simulink model "voicechanger"  (R2013a)
settings: Solver=ode45  StartTime=0.0  StopTime=10.0  RelTol=1e-3
libraries: dspxfrm3 x2, dspsrcs4 x1, commfilt2 x1, dspsnks4 x1
settings Model: Creator=Kevin  LastModifiedBy=Kevin

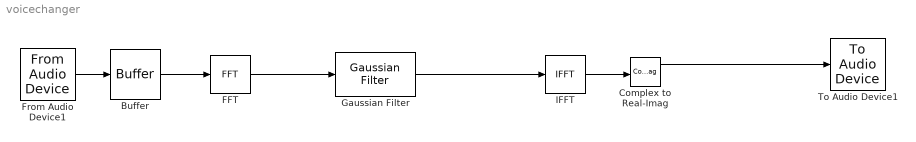
== system voicechanger ==
  Buffer : Buffer  N=100
  Complex to Real-Imag : ComplexToRealImag
  FFT : dspxfrm3/FFT  CompMethod=Table lookup  TableOpt=NEW  TableOptActive=Speed  BitRevOrder=off  InheritFFTLength=on  FFTLength=64  RowConvenienceOn=on  FFTImplementation=Auto  SkipNorm=off  firstCoeffDataTypeStr=Inherit: Same word length as input  firstCoeffLastDataTypeStr=Inherit: Same word length as input  outputMin=[]  outputMax=[]  roundingMode=Floor  overflowMode=off
  From Audio Device1 : dspsrcs4/From Audio Device  deviceName=主要音效擷取驅動程式  numChannels=1  sampleRate=44100  deviceDatatype=16-bit integer  autoBufferSize=on  bufferSize=4096  queueDuration=1.0  frameSize=500  outputDatatype=double
  Gaussian Filter : commfilt2/Gaussian Filter  N=8  BT=0.3  D=2  sampMode=Frame-based  normMode=Sum of coefficients  filterGain=1  checkCoeff=off  variableName=gaussFilt  launchFVT=off  roundingMode=Floor  overflowMode=off  InputProcessing=Columns as channels (frame based)
  IFFT : dspxfrm3/IFFT  CompMethod=Table lookup  TableOpt=NEW  TableOptActive=Speed  BitRevOrder=off  cs_in=off  SkipNorm=on  InheritFFTLength=on  FFTLength=64  mode=Complex  outSamplingMode=Sample based  RowConvenienceOn=on  FFTImplementation=Auto  firstCoeffDataTypeStr=Inherit: Same word length as input  firstCoeffLastDataTypeStr=Inherit: Same word length as input  outputMin=[]  outputMax=[]  roundingMode=Floor  overflowMode=off
  To Audio Device1 : dspsnks4/To Audio Device  deviceName=Default  inheritSampleRate=on  sampleRate=44100  deviceDatatype=Determine from input data type  autoBufferSize=on  bufferSize=4096  queueDuration=1.0
  wires:
  From Audio Device1/1 -> Buffer/1
  Buffer/1 -> FFT/1
  IFFT/1 -> Complex to Real-Imag/1
  Complex to Real-Imag/1 -> To Audio Device1/1
  FFT/1 -> Gaussian Filter/1
  Gaussian Filter/1 -> IFFT/1
